simulink model "Gas_Turbine_Model"  (Simulink 9.2)
settings: Solver=ode23s  StartTime=0.0  StopTime=500  FixedStep=0.001  RelTol=1e-3  EnableMultiTasking=on
values from neighbouring files (symbols this model uses):
  Beta_cmp = [1 1.5 2 2.5 3 3.5 4 4.5 5 5.5 6 6.5 ... (39 elements, 39x1)]    [Compressor_Map.mat]
  Eps_turb = [1 1.1 1.2 1.3 1.4 1.5 1.6 1.7 1.8 1.9 2 2.1 ... (191 elements, 1x191)]    [Turbine_Map.mat]
  Eta_cmp = [0.3 0.3 0.3 0.3 0.3 0.3 0.3 0.3 0.3 0.3 0.3 0.3 ... (585 elements, 15x39)]    [Compressor_Map.mat]
  Eta_turb = [0.586812592498 0.603057586725 0.61630240991 0.627098016156 0.635894182286 0.643058088048 0.648889484257 0.653633075447 0.657488628582 0.660619225395 0.663157999268 0.665213634952 ... (191 elements, 1x191)]    [Turbine_Map.mat]
  Mf_cmp = [0.246355651063 0.246355651063 0.246355651063 0.545009157509 1.57043960559 2.28211167924 2.75423550256 3.06528661824 3.27199659823 3.41123925415 3.50631480113 3.5719685441 ... (585 elements, 15x39)]    [Compressor_Map.mat]
  Mf_turb = [1.2124442703 1.39720469175 1.56286841441 1.71140925877 1.84459703271 1.96401861808 2.07109687783 2.16710760884 2.25319474261 2.3303839747 2.39959498557 2.4616523982 ... (191 elements, 1x191)]    [Turbine_Map.mat]
  N_cmp = [30000 35000 40000 45000 50000 55000 60000 65000 70000 75000 80000 85000 ... (15 elements, 1x15)]    [Compressor_Map.mat]
  pow_data = [49.5930192012 49.5930192012 47.1446947685 44.6063090759 42.0564349089 41.1061528351 40.7107031585 40.3152534819 41.8635649412 43.5549903366 45.246415732 45.7100796532 ... (145 elements, 1x145)]    [Pow_demand.mat]
  time_data = [0 600 1200 1800 2400 3000 3600 4200 4800 5400 6000 6600 ... (145 elements, 1x145)]    [Pow_demand.mat]
undefined symbols (not defined in the file or in its folder): cp, lambda, pamb, Tamb
settings Model: Creator=Xinmin Zhang  LastModifiedBy=canova.1
settings SolverCC: ZeroCrossAlgorithm=Adaptive
settings OptimizationCC: ExpressionDepthLimit=2147483647
settings DebuggingCC: AlgebraicLoopMsg=error  SolverPrmCheckMsg=warning

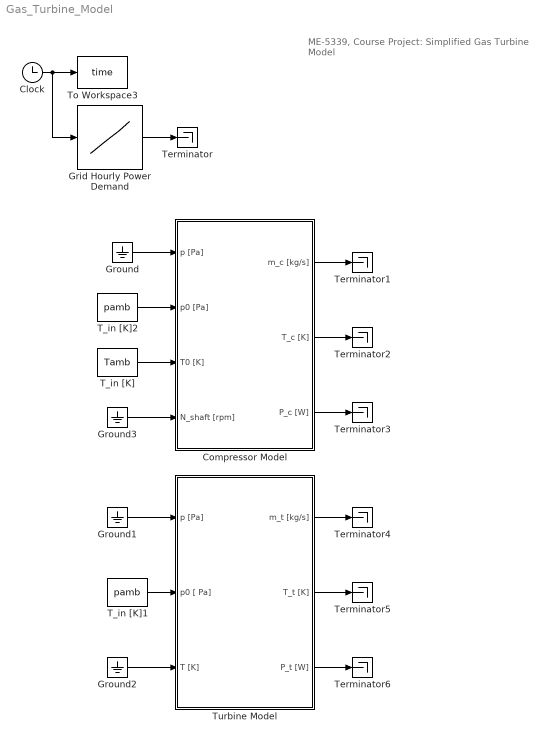
== system Gas_Turbine_Model ==
  note: ME-5339, Course Project:
      | Simplified Gas Turbine Model
  Clock : Clock
  Compressor Model : Subsystem
      mask help: Model of centrifugal compressor
  Grid Hourly Power Demand : Lookup_n-D  NumberOfTableDimensions=1  BreakpointsForDimension1=time_data  Table=pow_data  RndMeth=Simplest  InputSameDT=on
  Ground{,1..3} (4 alike) : Ground
  T_in [K] : Constant  Value=Tamb
  T_in [K]1 : Constant  Value=pamb
  T_in [K]2 : Constant  Value=pamb
  Terminator{,1..6} (7 alike) : Terminator
  To Workspace3 : ToWorkspace  VariableName=time  SampleTime=-1
  Turbine Model : Subsystem
      mask help: Model of radial inflow turbine
  wires:
  Clock/1 -> To Workspace3/1, Grid Hourly Power Demand/1
  T_in [K]2/1 -> Compressor Model/2(p0 [Pa])
  T_in [K]/1 -> Compressor Model/3(T0 [K])
  Grid Hourly Power Demand/1 -> Terminator/1
  Ground/1 -> Compressor Model/1(p [Pa])
  Ground1/1 -> Turbine Model/1(p [Pa])
  T_in [K]1/1 -> Turbine Model/2(p0 [ Pa])
  Ground2/1 -> Turbine Model/3(T [K])
  Compressor Model/1(m_c [kg/s]) -> Terminator1/1
  Compressor Model/2(T_c [K]) -> Terminator2/1
  Compressor Model/3(P_c [W]) -> Terminator3/1
  Turbine Model/1(m_t [kg/s]) -> Terminator4/1
  Turbine Model/2(T_t [K]) -> Terminator5/1
  Turbine Model/3(P_t [W]) -> Terminator6/1
  Ground3/1 -> Compressor Model/4(N_shaft [rpm])

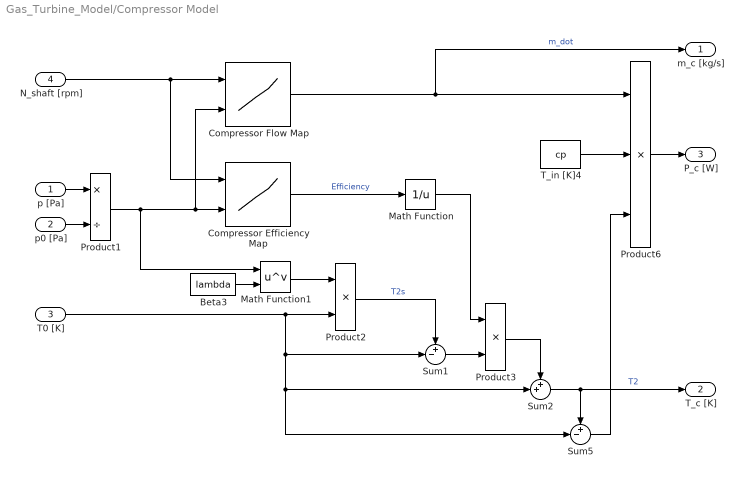
== system Gas_Turbine_Model/Compressor Model ==
  p [Pa] : Inport
  p0 [Pa] : Inport  Port=2
  T0 [K] : Inport  Port=3
  N_shaft [rpm] : Inport  Port=4
  Beta3 : Constant  Value=lambda
  Compressor Efficiency Map : Lookup_n-D  BreakpointsForDimension1=N_cmp  BreakpointsForDimension2=Beta_cmp  Table=Eta_cmp  RndMeth=Simplest  InputSameDT=on
  Compressor Flow Map : Lookup_n-D  BreakpointsForDimension1=N_cmp  BreakpointsForDimension2=Beta_cmp  Table=Mf_cmp  RndMeth=Simplest  InputSameDT=on
  Math Function : Math  Operator=reciprocal  SaturateOnIntegerOverflow=on
  Math Function1 : Math  Operator=pow  SaturateOnIntegerOverflow=on
  Product1 : Product  Inputs=*/  RndMeth=Zero
  Product2 : Product  RndMeth=Zero
  Product3 : Product  RndMeth=Zero
  Product6 : Product  Inputs=3  RndMeth=Zero
  Sum1 : Sum  Inputs=+-|
  Sum2 : Sum  Inputs=++|
  Sum5 : Sum  Inputs=+-|
  T_in [K]4 : Constant  Value=cp
  m_c [kg/s] : Outport
  T_c [K] : Outport  Port=2
  P_c [W] : Outport  Port=3
  wires:
  N_shaft [rpm]/1 -> Compressor Efficiency Map/1, Compressor Flow Map/1
  Product1/1 -> Compressor Efficiency Map/2, Compressor Flow Map/2, Math Function1/1
  Compressor Efficiency Map/1 -> Math Function/1  "Efficiency"
  Beta3/1 -> Math Function1/2
  Math Function1/1 -> Product2/1
  Product2/1 -> Sum1/1  "T2s"
  T0 [K]/1 -> Sum1/2, Sum2/2, Sum5/2, Product2/2
  Sum1/1 -> Product3/2
  Math Function/1 -> Product3/1
  Product3/1 -> Sum2/1
  Compressor Flow Map/1 -> m_c [kg/s]/1, Product6/1  "m_dot"
  p [Pa]/1 -> Product1/1
  p0 [Pa]/1 -> Product1/2
  Sum2/1 -> T_c [K]/1, Sum5/1  "T2"
  Product6/1 -> P_c [W]/1
  T_in [K]4/1 -> Product6/2
  Sum5/1 -> Product6/3

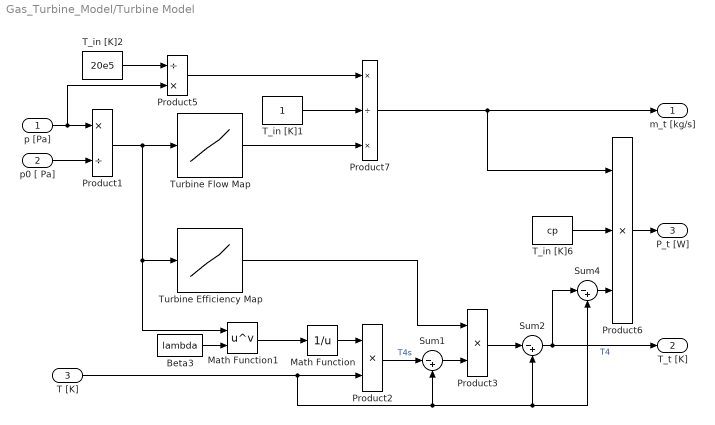
== system Gas_Turbine_Model/Turbine Model ==
  p [Pa] : Inport
  p0 [ Pa] : Inport  Port=2
  T [K] : Inport  Port=3
  Beta3 : Constant  Value=lambda
  Math Function : Math  Operator=reciprocal  SaturateOnIntegerOverflow=on
  Math Function1 : Math  Operator=pow  SaturateOnIntegerOverflow=on
  Product1 : Product  Inputs=*/  RndMeth=Zero
  Product2 : Product  RndMeth=Zero
  Product3 : Product  RndMeth=Zero
  Product5 : Product  Inputs=/*  RndMeth=Zero
  Product6 : Product  Inputs=3  RndMeth=Zero
  Product7 : Product  Inputs=*/*  RndMeth=Zero
  Sum1 : Sum  Inputs=|-+
  Sum2 : Sum  Inputs=|-+
  Sum4 : Sum  Inputs=|-+
  T_in [K]1 : Constant
  T_in [K]2 : Constant  Value=20e5
  T_in [K]6 : Constant  Value=cp
  Turbine Efficiency Map : Lookup_n-D  NumberOfTableDimensions=1  BreakpointsForDimension1=Eps_turb  Table=Eta_turb  RndMeth=Simplest  InputSameDT=on
  Turbine Flow Map : Lookup_n-D  NumberOfTableDimensions=1  BreakpointsForDimension1=Eps_turb  Table=Mf_turb  RndMeth=Simplest  InputSameDT=on
  m_t [kg/s] : Outport
  T_t [K] : Outport  Port=2
  P_t [W] : Outport  Port=3
  wires:
  Beta3/1 -> Math Function1/2
  Math Function1/1 -> Math Function/1
  T [K]/1 -> Sum4/2, Sum2/2, Sum1/2, Product2/2
  Math Function/1 -> Product2/1
  Product2/1 -> Sum1/1  "T4s"
  Sum1/1 -> Product3/2
  Product3/1 -> Sum2/1
  Sum2/1 -> Sum4/1, T_t [K]/1  "T4"
  T_in [K]6/1 -> Product6/2
  Sum4/1 -> Product6/3
  Turbine Efficiency Map/1 -> Product3/1
  Product6/1 -> P_t [W]/1
  Product1/1 -> Turbine Flow Map/1, Turbine Efficiency Map/1, Math Function1/1
  Turbine Flow Map/1 -> Product7/3
  T_in [K]2/1 -> Product5/1
  Product5/1 -> Product7/1
  T_in [K]1/1 -> Product7/2
  Product7/1 -> m_t [kg/s]/1, Product6/1
  p [Pa]/1 -> Product1/1, Product5/2
  p0 [ Pa]/1 -> Product1/2
